simulink model "Scenario_3"  (R2020b)
settings: Solver=ode1  StartTime=0.0  StopTime=10.0  RelTol=1e-3
InitFcn:
  | Scenario_3_parameters;
values from neighbouring files (symbols this model uses):
  c0 = c0_zeb    (= 6.57988e-09)    [Scenario_17_parameters.m]    (also in Scenario_1_parameters.m = 6.37282e-09; Scenario_2_parameters.m = 6.37282e-09; Scenario_3_parameters.m)
  c0_hawk = 6.37282e-09    [Scenario_17_parameters.m]    (also in Scenario_1_parameters.m; Scenario_2_parameters.m; Scenario_3_parameters.m)
  c1 = c1_zeb    (= 9.15905e-09)    [Scenario_17_parameters.m]    (also in Scenario_1_parameters.m = 8.76156e-09; Scenario_2_parameters.m = 8.76156e-09; Scenario_3_parameters.m)
  c1_hawk = 8.76156e-09    [Scenario_17_parameters.m]    (also in Scenario_1_parameters.m; Scenario_2_parameters.m; Scenario_3_parameters.m)
  fg = 50    [Scenario_17_parameters.m]    (also in Scenario_1_parameters.m; Scenario_2_parameters.m; Scenario_3_parameters.m)
  G10gen = 0.85    [Scenario_3_parameters.m]
  G12gen = 0.85    [Scenario_3_parameters.m]
  G1gen = 0.50    (= 0.5)    [Scenario_17_parameters.m]    (also in Scenario_1_parameters.m = 0.2; Scenario_2_parameters.m = 0.1245; Scenario_3_parameters.m = 0.45)
  G2gen = 0.30    (= 0.3)    [Scenario_1_parameters.m]    (also in Scenario_2_parameters.m; Scenario_3_parameters.m = 0.4)
  G3gen = 0.25    [Scenario_1_parameters.m]    (also in Scenario_2_parameters.m = 0.2; Scenario_3_parameters.m = 0.6)
  G4gen = 0.95    [Scenario_3_parameters.m]
  G5gen = 0.75    [Scenario_17_parameters.m]    (also in Scenario_1_parameters.m = 0.22; Scenario_2_parameters.m = 0.2; Scenario_3_parameters.m = 0.7)
  G6gen = 0.90    (= 0.9)    [Scenario_17_parameters.m]    (also in Scenario_1_parameters.m = 0.41; Scenario_2_parameters.m = 0.2078; Scenario_3_parameters.m = 0.95)
  G7gen = 0.60    (= 0.6)    [Scenario_17_parameters.m]    (also in Scenario_1_parameters.m = 0.52; Scenario_2_parameters.m = 0.518; Scenario_3_parameters.m = 0.5)
  G8gen = 0.55    [Scenario_17_parameters.m]    (also in Scenario_3_parameters.m = 0.65)
  G9gen = 0.85    [Scenario_17_parameters.m]    (also in Scenario_3_parameters.m = 0.75)
  Ihvpk = Ihv*sqrt(2)    [Scenario_17_parameters.m]    (also in Scenario_1_parameters.m; Scenario_2_parameters.m; Scenario_3_parameters.m)
  l0 = l0_zeb    (= 0.00368)    [Scenario_17_parameters.m]    (also in Scenario_1_parameters.m = 0.00373; Scenario_2_parameters.m = 0.00373; Scenario_3_parameters.m)
  l0_hawk = 0.00373    [Scenario_17_parameters.m]    (also in Scenario_1_parameters.m; Scenario_2_parameters.m; Scenario_3_parameters.m)
  l1 = l1_zeb    (= 0.00128)    [Scenario_17_parameters.m]    (also in Scenario_1_parameters.m = 0.00133; Scenario_2_parameters.m = 0.00133; Scenario_3_parameters.m)
  L10dem = 0.10    (= 0.1)    [Scenario_3_parameters.m]
  L12dem = 0.025    [Scenario_17_parameters.m]    (also in Scenario_3_parameters.m = 0.005)
  L13dem = 0.005    [Scenario_3_parameters.m]
  l1_hawk = 0.00133    [Scenario_17_parameters.m]    (also in Scenario_1_parameters.m; Scenario_2_parameters.m; Scenario_3_parameters.m)
  L1dem = 0.25    [Scenario_17_parameters.m]    (also in Scenario_3_parameters.m = 0.1)
  L3dem = 0.30    (= 0.3)    [Scenario_17_parameters.m]    (also in Scenario_1_parameters.m = 0.1; Scenario_2_parameters.m = 0.1; Scenario_3_parameters.m = 0.2)
  L6dem = 0.15    [Scenario_1_parameters.m]    (also in Scenario_2_parameters.m; Scenario_3_parameters.m = 0.1)
  L7dem = 0.10    (= 0.1)    [Scenario_1_parameters.m]    (also in Scenario_2_parameters.m; Scenario_3_parameters.m = 0.15)
  L9dem = 0.15    [Scenario_17_parameters.m]    (also in Scenario_3_parameters.m)
  Pr = Sr*PF    (= 1900000000)    [Scenario_17_parameters.m]    (also in Scenario_1_parameters.m = 550050000; Scenario_2_parameters.m = 550050000; Scenario_3_parameters.m = 11640000000)
  Qr = sqrt(Sr^2 - Pr^2)    [Scenario_17_parameters.m]    (also in Scenario_1_parameters.m; Scenario_2_parameters.m; Scenario_3_parameters.m)
  r0 = r0_zeb    (= 0.39362)    [Scenario_17_parameters.m]    (also in Scenario_1_parameters.m = 0.44587; Scenario_2_parameters.m = 0.44587; Scenario_3_parameters.m)
  r0_hawk = 0.44587    [Scenario_17_parameters.m]    (also in Scenario_1_parameters.m; Scenario_2_parameters.m; Scenario_3_parameters.m)
  r1 = r1_zeb    (= 0.06862)    [Scenario_17_parameters.m]    (also in Scenario_1_parameters.m = 0.12087; Scenario_2_parameters.m = 0.12087; Scenario_3_parameters.m)
  r1_hawk = 0.12087    [Scenario_17_parameters.m]    (also in Scenario_1_parameters.m; Scenario_2_parameters.m; Scenario_3_parameters.m)
  Rtpu = Xtpu/40    (= 0.0025)    [Scenario_17_parameters.m]    (also in Scenario_1_parameters.m = 0.00375; Scenario_2_parameters.m = 0.00375; Scenario_3_parameters.m = 0.00375)
  S10non = 500e6    (= 500000000)    [Scenario_3_parameters.m]
  S12non = 1500e6    (= 1500000000)    [Scenario_3_parameters.m]
  S1non = 700e6    (= 700000000)    [Scenario_17_parameters.m]    (also in Scenario_1_parameters.m = 400000000; Scenario_2_parameters.m = 400000000; Scenario_3_parameters.m = 1000000000)
  S2non = 300e6    (= 300000000)    [Scenario_1_parameters.m]    (also in Scenario_2_parameters.m; Scenario_3_parameters.m = 3000000000)
  S3non = 200e6    (= 200000000)    [Scenario_1_parameters.m]    (also in Scenario_2_parameters.m; Scenario_3_parameters.m = 1000000000)
  S4non = 2000e6    (= 2000000000)    [Scenario_3_parameters.m]
  S5non = 400e6    (= 400000000)    [Scenario_17_parameters.m]    (also in Scenario_1_parameters.m = 500000000; Scenario_2_parameters.m = 500000000; Scenario_3_parameters.m = 2000000000)
  S6non = 150e6    (= 150000000)    [Scenario_17_parameters.m]    (also in Scenario_1_parameters.m = 400000000; Scenario_2_parameters.m = 400000000; Scenario_3_parameters.m = 3000000000)
  S7non = 1000e6    (= 1000000000)    [Scenario_17_parameters.m]    (also in Scenario_1_parameters.m = 200000000; Scenario_2_parameters.m = 200000000; Scenario_3_parameters.m = 4000000000)
  S8non = 600e6    (= 600000000)    [Scenario_17_parameters.m]    (also in Scenario_3_parameters.m = 2000000000)
  S9non = 200e6    (= 200000000)    [Scenario_17_parameters.m]    (also in Scenario_3_parameters.m = 1500000000)
  tonvsc = 0.01    [Scenario_17_parameters.m]    (also in Scenario_1_parameters.m = 0.02; Scenario_2_parameters.m; Scenario_3_parameters.m = 0.05)
  Ts = 100e-6    (= 0.0001)    [Scenario_17_parameters.m]    (also in Scenario_1_parameters.m; Scenario_2_parameters.m; Scenario_3_parameters.m = 5e-05)
  Vhv = 220e3    (= 220000)    [Scenario_17_parameters.m]    (also in Scenario_1_parameters.m; Scenario_2_parameters.m; Scenario_3_parameters.m)
  Vmv = 22e3    (= 22000)    [Scenario_17_parameters.m]    (also in Scenario_1_parameters.m; Scenario_2_parameters.m; Scenario_3_parameters.m)
  wc1 = wsw1/10    (= 848.230016469)    [Scenario_17_parameters.m]    (also in Scenario_1_parameters.m; Scenario_2_parameters.m; Scenario_3_parameters.m)
  wdc1 = wc1/10    (= 84.8230016469)    [Scenario_17_parameters.m]    (also in Scenario_1_parameters.m; Scenario_2_parameters.m; Scenario_3_parameters.m)
  wpq1 = wc1/10    (= 84.8230016469)    [Scenario_17_parameters.m]    (also in Scenario_1_parameters.m; Scenario_2_parameters.m; Scenario_3_parameters.m)
  wsw1 = ksw1*2*pi*fg    (= 8482.30016469)    [Scenario_17_parameters.m]    (also in Scenario_1_parameters.m; Scenario_2_parameters.m; Scenario_3_parameters.m)
  Xtpu = 0.10    (= 0.1)    [Scenario_17_parameters.m]    (also in Scenario_1_parameters.m = 0.15; Scenario_2_parameters.m = 0.15; Scenario_3_parameters.m = 0.15)
undefined symbols (not defined in the file or in its folder): D11, Delta, Kf, r, theta0
libraries: powerlib x426, simulink_extras x305, powerlib_meascontrol x139, pid_lib x109, eeGeneralControl x72, simulink x60, eeTransforms x54, spsFirstOrderFilterLib x36, eePwmGeneratorTwoLevel x9
(part 8 of 36)

== system Scenario_3/G10/VSC/VI measurement ==
  Current Measurement : powerlib/Measurements/Current Measurement  PhasorSimulation=on  OutputType=Complex  PSBequivalent=0
  Current Measurement1 : powerlib/Measurements/Current Measurement  PhasorSimulation=on  OutputType=Complex  PSBequivalent=0
  Current Measurement2 : powerlib/Measurements/Current Measurement  PhasorSimulation=on  OutputType=Complex  PSBequivalent=0
  Ground : powerlib/Elements/Ground  LConnTagsString=a
  Ground1 : powerlib/Elements/Ground  LConnTagsString=a
  Ground2 : powerlib/Elements/Ground  LConnTagsString=a
  Mux : Mux  Inputs=3
  Mux1 : Mux  Inputs=3
  Voltage Measurement : powerlib/Measurements/Voltage Measurement  PhasorSimulation=on  OutputType=Complex  PSBequivalent=0
  Voltage Measurement1 : powerlib/Measurements/Voltage Measurement  PhasorSimulation=on  OutputType=Complex  PSBequivalent=0
  Voltage Measurement2 : powerlib/Measurements/Voltage Measurement  PhasorSimulation=on  OutputType=Complex  PSBequivalent=0
  A : PMIOPort  Side=Left
  B : PMIOPort  Port=2  Side=Left
  C : PMIOPort  Port=3  Side=Left
  a : PMIOPort  Port=4  Side=Right
  b : PMIOPort  Port=5  Side=Right
  c : PMIOPort  Port=6  Side=Right
  Vs : Outport
  Is : Outport  Port=2
  wires:
  Mux1/1 -> Is/1
  Mux/1 -> Vs/1
  Voltage Measurement1/1 -> Mux/2
  Voltage Measurement2/1 -> Mux/3
  Current Measurement2/1 -> Mux1/3
  Voltage Measurement/1 -> Mux/1
  Current Measurement/1 -> Mux1/1
  Current Measurement1/1 -> Mux1/2
  connections:
  Voltage Measurement/LConn1 -- Current Measurement/LConn1 -- A/RConn1
  Current Measurement2/LConn1 -- C/RConn1 -- Voltage Measurement2/LConn1
  Current Measurement1/LConn1 -- Voltage Measurement1/LConn1 -- B/RConn1
  Current Measurement1/RConn1 -- b/RConn1
  Current Measurement/RConn1 -- a/RConn1
  Ground/LConn1 -- Voltage Measurement/LConn2
  Current Measurement2/RConn1 -- c/RConn1
  Ground1/LConn1 -- Voltage Measurement1/LConn2
  Ground2/LConn1 -- Voltage Measurement2/LConn2

== system Scenario_3/G10/VSC/VSC Control ==
  Block : Inport
  Vabc : Inport  Port=2
  Iabc : Inport  Port=3
  Pset : Inport  Port=4
  Qset : Inport  Port=5
  Control loops : Subsystem  Variant=on  VariantControlMode=label  LabelModeActiveChoice=Phasor_I_ref
  Measurements : Subsystem  Variant=on  VariantControlMode=label  LabelModeActiveChoice=Phasor
  Modulation : Subsystem  Variant=on  VariantControlMode=label  LabelModeActiveChoice=Phasor_I_and_PQ
  Mux : Mux  Inputs=2
  Ref : Outport
  m : Outport  Port=2
  wires:
  Control loops/2(iqd+-ref) -> Modulation/3(iqd+-*)
  Control loops/1(vqd+-ref) -> Modulation/2(vqd+-*)
  [PQabc] -> Mux/2
  Measurements/5(PQabc) -> [PQabc]
  Modulation/1(Ref) -> Ref/1
  Measurements/4(theta) -> [theta]
  Vabc/1 -> Measurements/1(Vabc)
  Measurements/1(vqd+-) -> Control loops/3(vqd+-), [vqdpn]
  Measurements/2(iqd+-) -> Control loops/4(iqd+-)
  Measurements/3(freq) -> Control loops/5(freq)
  [theta] -> Modulation/4(theta)
  [vqdpn] -> Modulation/1(vqd+-)
  Iabc/1 -> Measurements/2(Iabc)
  Mux/1 -> m/1
  Control loops/3(m) -> Mux/1
  Pset/1 -> Control loops/1(Pset)
  Qset/1 -> Control loops/2(Qset)
  Block/1 -> Control loops/6(Block)

== system Scenario_3/G10/VSC/VSC Model ==
  Ref : Inport
  EMT AVG : Subsystem  VariantControl=EMT_AVG
      settings: PortSchema="{\"entries\":[{\"content\":{\"sides\":[{\"content\":{\"connectorIds\":[\"LConn1\",\"LConn2\",\"LConn3\"]},\"type\":\"ConnectorPlacement.EquallySpacedRectSide\",\"uuid\":\"96043b84-a665-4cb2-a938-d6633d7ee474\"},{\"content\":{\"connectorIds\":[\"In1\"],\"side\":\"RIGHT\"},\"type\":\"ConnectorPlacement.EquallySpacedRectSide\",\"uuid\":\"064d463f-c23a-42ac-89ce-8dea3d446214\"},{\"content\":{\"connectorIds\":[],\"side\":\"TOP\"},\"type\":\"ConnectorPlacement.EquallySpacedRectSide\",\"uuid\":\"95ef669c-c6ed-44c3-8b69-447906728b6d\"}]},\"type\":\"ConnectorPlacement.EquallySpacedConnector\",\"uuid\":\"ea66db09-64d7-4d7e-ba7b-d769c56e2dbd\"}],\"packageUris\":[\"http://schema.mathworks.com/mf0/Connector/19700101\"],\"version\":\"1.0\"}"
  EMT SW : Subsystem  VariantControl=EMT_SW
      settings: PortSchema="{\"entries\":[{\"content\":{\"sides\":[{\"content\":{\"connectorIds\":[\"LConn1\",\"LConn2\",\"LConn3\"]},\"type\":\"ConnectorPlacement.EquallySpacedRectSide\",\"uuid\":\"96043b84-a665-4cb2-a938-d6633d7ee474\"},{\"content\":{\"connectorIds\":[\"In1\"],\"side\":\"RIGHT\"},\"type\":\"ConnectorPlacement.EquallySpacedRectSide\",\"uuid\":\"064d463f-c23a-42ac-89ce-8dea3d446214\"},{\"content\":{\"connectorIds\":[],\"side\":\"TOP\"},\"type\":\"ConnectorPlacement.EquallySpacedRectSide\",\"uuid\":\"95ef669c-c6ed-44c3-8b69-447906728b6d\"}]},\"type\":\"ConnectorPlacement.EquallySpacedConnector\",\"uuid\":\"ea66db09-64d7-4d7e-ba7b-d769c56e2dbd\"}],\"packageUris\":[\"http://schema.mathworks.com/mf0/Connector/19700101\"],\"version\":\"1.0\"}"
  Phasor : Subsystem  VariantControl=Phasor
      settings: PortSchema="{\"entries\":[{\"content\":{\"sides\":[{\"content\":{\"connectorIds\":[\"LConn1\",\"LConn2\",\"LConn3\"]},\"type\":\"ConnectorPlacement.EquallySpacedRectSide\",\"uuid\":\"96043b84-a665-4cb2-a938-d6633d7ee474\"},{\"content\":{\"connectorIds\":[\"In1\"],\"side\":\"RIGHT\"},\"type\":\"ConnectorPlacement.EquallySpacedRectSide\",\"uuid\":\"064d463f-c23a-42ac-89ce-8dea3d446214\"},{\"content\":{\"connectorIds\":[],\"side\":\"TOP\"},\"type\":\"ConnectorPlacement.EquallySpacedRectSide\",\"uuid\":\"95ef669c-c6ed-44c3-8b69-447906728b6d\"}]},\"type\":\"ConnectorPlacement.EquallySpacedConnector\",\"uuid\":\"ea66db09-64d7-4d7e-ba7b-d769c56e2dbd\"}],\"packageUris\":[\"http://schema.mathworks.com/mf0/Connector/19700101\"],\"version\":\"1.0\"}"
  A : PMIOPort  Side=Left
  B : PMIOPort  Port=2  Side=Left
  C : PMIOPort  Port=3  Side=Left

== system Scenario_3/G10/VSC/output signals ==
  Vs : Inport
  Is : Inport  Port=2
  control : Inport  Port=3
  Bus Creator : BusCreator  Inputs=15
  Demux : Demux  Outputs=13
  m : Outport
  wires:
  Bus Creator/1 -> m/1
  control/1 -> Demux/1
  Vs/1 -> Bus Creator/1  "Vabc"
  Is/1 -> Bus Creator/2  "Iabc"
  Demux/1 -> Bus Creator/3  "vqp"
  Demux/2 -> Bus Creator/4  "vdp"
  Demux/3 -> Bus Creator/5  "vqn"
  Demux/4 -> Bus Creator/6  "vdn"
  Demux/5 -> Bus Creator/7  "iqp"
  Demux/6 -> Bus Creator/8  "idp"
  Demux/7 -> Bus Creator/9  "iqn"
  Demux/8 -> Bus Creator/10  "idn"
  Demux/9 -> Bus Creator/11  "f"
  Demux/10 -> Bus Creator/12  "Pdq"
  Demux/11 -> Bus Creator/13  "Qdq"
  Demux/12 -> Bus Creator/14  "Pabc"
  Demux/13 -> Bus Creator/15  "Qabc"

== system Scenario_3/G12/VSC/VI measurement ==
  Current Measurement : powerlib/Measurements/Current Measurement  PhasorSimulation=on  OutputType=Complex  PSBequivalent=0
  Current Measurement1 : powerlib/Measurements/Current Measurement  PhasorSimulation=on  OutputType=Complex  PSBequivalent=0
  Current Measurement2 : powerlib/Measurements/Current Measurement  PhasorSimulation=on  OutputType=Complex  PSBequivalent=0
  Ground : powerlib/Elements/Ground  LConnTagsString=a
  Ground1 : powerlib/Elements/Ground  LConnTagsString=a
  Ground2 : powerlib/Elements/Ground  LConnTagsString=a
  Mux : Mux  Inputs=3
  Mux1 : Mux  Inputs=3
  Voltage Measurement : powerlib/Measurements/Voltage Measurement  PhasorSimulation=on  OutputType=Complex  PSBequivalent=0
  Voltage Measurement1 : powerlib/Measurements/Voltage Measurement  PhasorSimulation=on  OutputType=Complex  PSBequivalent=0
  Voltage Measurement2 : powerlib/Measurements/Voltage Measurement  PhasorSimulation=on  OutputType=Complex  PSBequivalent=0
  A : PMIOPort  Side=Left
  B : PMIOPort  Port=2  Side=Left
  C : PMIOPort  Port=3  Side=Left
  a : PMIOPort  Port=4  Side=Right
  b : PMIOPort  Port=5  Side=Right
  c : PMIOPort  Port=6  Side=Right
  Vs : Outport
  Is : Outport  Port=2
  wires:
  Mux1/1 -> Is/1
  Mux/1 -> Vs/1
  Voltage Measurement1/1 -> Mux/2
  Voltage Measurement2/1 -> Mux/3
  Current Measurement2/1 -> Mux1/3
  Voltage Measurement/1 -> Mux/1
  Current Measurement/1 -> Mux1/1
  Current Measurement1/1 -> Mux1/2
  connections:
  Voltage Measurement/LConn1 -- Current Measurement/LConn1 -- A/RConn1
  Current Measurement2/LConn1 -- C/RConn1 -- Voltage Measurement2/LConn1
  Current Measurement1/LConn1 -- Voltage Measurement1/LConn1 -- B/RConn1
  Current Measurement1/RConn1 -- b/RConn1
  Current Measurement/RConn1 -- a/RConn1
  Ground/LConn1 -- Voltage Measurement/LConn2
  Current Measurement2/RConn1 -- c/RConn1
  Ground1/LConn1 -- Voltage Measurement1/LConn2
  Ground2/LConn1 -- Voltage Measurement2/LConn2

== system Scenario_3/G12/VSC/VSC Control ==
  Block : Inport
  Vabc : Inport  Port=2
  Iabc : Inport  Port=3
  Pset : Inport  Port=4
  Qset : Inport  Port=5
  Control loops : Subsystem  Variant=on  VariantControlMode=label  LabelModeActiveChoice=Phasor_I_ref
  Measurements : Subsystem  Variant=on  VariantControlMode=label  LabelModeActiveChoice=Phasor
  Modulation : Subsystem  Variant=on  VariantControlMode=label  LabelModeActiveChoice=Phasor_I_and_PQ
  Mux : Mux  Inputs=2
  Ref : Outport
  m : Outport  Port=2
  wires:
  Control loops/2(iqd+-ref) -> Modulation/3(iqd+-*)
  Control loops/1(vqd+-ref) -> Modulation/2(vqd+-*)
  [PQabc] -> Mux/2
  Measurements/5(PQabc) -> [PQabc]
  Modulation/1(Ref) -> Ref/1
  Measurements/4(theta) -> [theta]
  Vabc/1 -> Measurements/1(Vabc)
  Measurements/1(vqd+-) -> Control loops/3(vqd+-), [vqdpn]
  Measurements/2(iqd+-) -> Control loops/4(iqd+-)
  Measurements/3(freq) -> Control loops/5(freq)
  [theta] -> Modulation/4(theta)
  [vqdpn] -> Modulation/1(vqd+-)
  Iabc/1 -> Measurements/2(Iabc)
  Mux/1 -> m/1
  Control loops/3(m) -> Mux/1
  Pset/1 -> Control loops/1(Pset)
  Qset/1 -> Control loops/2(Qset)
  Block/1 -> Control loops/6(Block)

== system Scenario_3/G12/VSC/VSC Model ==
  Ref : Inport
  EMT AVG : Subsystem  VariantControl=EMT_AVG
      settings: PortSchema="{\"entries\":[{\"content\":{\"sides\":[{\"content\":{\"connectorIds\":[\"LConn1\",\"LConn2\",\"LConn3\"]},\"type\":\"ConnectorPlacement.EquallySpacedRectSide\",\"uuid\":\"96043b84-a665-4cb2-a938-d6633d7ee474\"},{\"content\":{\"connectorIds\":[\"In1\"],\"side\":\"RIGHT\"},\"type\":\"ConnectorPlacement.EquallySpacedRectSide\",\"uuid\":\"064d463f-c23a-42ac-89ce-8dea3d446214\"},{\"content\":{\"connectorIds\":[],\"side\":\"TOP\"},\"type\":\"ConnectorPlacement.EquallySpacedRectSide\",\"uuid\":\"95ef669c-c6ed-44c3-8b69-447906728b6d\"}]},\"type\":\"ConnectorPlacement.EquallySpacedConnector\",\"uuid\":\"ea66db09-64d7-4d7e-ba7b-d769c56e2dbd\"}],\"packageUris\":[\"http://schema.mathworks.com/mf0/Connector/19700101\"],\"version\":\"1.0\"}"
  EMT SW : Subsystem  VariantControl=EMT_SW
      settings: PortSchema="{\"entries\":[{\"content\":{\"sides\":[{\"content\":{\"connectorIds\":[\"LConn1\",\"LConn2\",\"LConn3\"]},\"type\":\"ConnectorPlacement.EquallySpacedRectSide\",\"uuid\":\"96043b84-a665-4cb2-a938-d6633d7ee474\"},{\"content\":{\"connectorIds\":[\"In1\"],\"side\":\"RIGHT\"},\"type\":\"ConnectorPlacement.EquallySpacedRectSide\",\"uuid\":\"064d463f-c23a-42ac-89ce-8dea3d446214\"},{\"content\":{\"connectorIds\":[],\"side\":\"TOP\"},\"type\":\"ConnectorPlacement.EquallySpacedRectSide\",\"uuid\":\"95ef669c-c6ed-44c3-8b69-447906728b6d\"}]},\"type\":\"ConnectorPlacement.EquallySpacedConnector\",\"uuid\":\"ea66db09-64d7-4d7e-ba7b-d769c56e2dbd\"}],\"packageUris\":[\"http://schema.mathworks.com/mf0/Connector/19700101\"],\"version\":\"1.0\"}"
  Phasor : Subsystem  VariantControl=Phasor
      settings: PortSchema="{\"entries\":[{\"content\":{\"sides\":[{\"content\":{\"connectorIds\":[\"LConn1\",\"LConn2\",\"LConn3\"]},\"type\":\"ConnectorPlacement.EquallySpacedRectSide\",\"uuid\":\"96043b84-a665-4cb2-a938-d6633d7ee474\"},{\"content\":{\"connectorIds\":[\"In1\"],\"side\":\"RIGHT\"},\"type\":\"ConnectorPlacement.EquallySpacedRectSide\",\"uuid\":\"064d463f-c23a-42ac-89ce-8dea3d446214\"},{\"content\":{\"connectorIds\":[],\"side\":\"TOP\"},\"type\":\"ConnectorPlacement.EquallySpacedRectSide\",\"uuid\":\"95ef669c-c6ed-44c3-8b69-447906728b6d\"}]},\"type\":\"ConnectorPlacement.EquallySpacedConnector\",\"uuid\":\"ea66db09-64d7-4d7e-ba7b-d769c56e2dbd\"}],\"packageUris\":[\"http://schema.mathworks.com/mf0/Connector/19700101\"],\"version\":\"1.0\"}"
  A : PMIOPort  Side=Left
  B : PMIOPort  Port=2  Side=Left
  C : PMIOPort  Port=3  Side=Left

== system Scenario_3/G12/VSC/output signals ==
  Vs : Inport
  Is : Inport  Port=2
  control : Inport  Port=3
  Bus Creator : BusCreator  Inputs=15
  Demux : Demux  Outputs=13
  m : Outport
  wires:
  Bus Creator/1 -> m/1
  control/1 -> Demux/1
  Vs/1 -> Bus Creator/1  "Vabc"
  Is/1 -> Bus Creator/2  "Iabc"
  Demux/1 -> Bus Creator/3  "vqp"
  Demux/2 -> Bus Creator/4  "vdp"
  Demux/3 -> Bus Creator/5  "vqn"
  Demux/4 -> Bus Creator/6  "vdn"
  Demux/5 -> Bus Creator/7  "iqp"
  Demux/6 -> Bus Creator/8  "idp"
  Demux/7 -> Bus Creator/9  "iqn"
  Demux/8 -> Bus Creator/10  "idn"
  Demux/9 -> Bus Creator/11  "f"
  Demux/10 -> Bus Creator/12  "Pdq"
  Demux/11 -> Bus Creator/13  "Qdq"
  Demux/12 -> Bus Creator/14  "Pabc"
  Demux/13 -> Bus Creator/15  "Qabc"

== system Scenario_3/G2/Exciter System/PSS ==
  note: Power System Stabilizer (PSS2A)
  dw : Inport
  Pgen : Inport  Port=2
  Gain : Gain  Gain=Ks1
  Gain1 : Gain  Gain=Ks3
  Saturation : Saturate  UpperLimit=Vstmax  LowerLimit=Vstmin
  Sum1 : Sum  Inputs=|++
  Sum2 : Sum  Inputs=|+-
  Transfer Fcn1 : TransferFcn  Numerator=[Tw1 0]  Denominator=[Tw1 1]
  Transfer Fcn2 : TransferFcn  Numerator=[Tw3 0]  Denominator=[Tw3 1]
  Transfer Fcn3 : TransferFcn  Numerator=[Tw2 0]  Denominator=[Tw2 1]
  Transfer Fcn4 : TransferFcn  Denominator=[T6 1]
  Transfer Fcn5 : TransferFcn  Numerator=[T8 1].^N  Denominator=[T9 1].^(M*N)
  Transfer Fcn6 : TransferFcn  Numerator=[T1 1]  Denominator=[T2 1]
  Transfer Fcn7 : TransferFcn  Numerator=[T3 1]  Denominator=[T4 1]
  Transfer Fcn8 : TransferFcn  Numerator=[Tw4 0]  Denominator=[Tw4 1]
  Transfer Fcn9 : TransferFcn  Numerator=[Ks2]  Denominator=[T7 1]
  Vothsg : Outport
  wires:
  Transfer Fcn9/1 -> Sum2/2, Gain1/1
  Gain1/1 -> Sum1/2
  Transfer Fcn8/1 -> Transfer Fcn9/1
  Transfer Fcn2/1 -> Transfer Fcn8/1
  Pgen/1 -> Transfer Fcn2/1
  Saturation/1 -> Vothsg/1
  Transfer Fcn7/1 -> Saturation/1
  Transfer Fcn6/1 -> Transfer Fcn7/1
  Gain/1 -> Transfer Fcn6/1
  Sum2/1 -> Gain/1
  Transfer Fcn5/1 -> Sum2/1
  Sum1/1 -> Transfer Fcn5/1
  Transfer Fcn4/1 -> Sum1/1
  Transfer Fcn3/1 -> Transfer Fcn4/1
  Transfer Fcn1/1 -> Transfer Fcn3/1
  dw/1 -> Transfer Fcn1/1

== system Scenario_3/G2/Exciter System/SEXS ==
  note: The controller parameters provided by ENTSO-E
      | define different names for the parameters:
      |
      | ENTSO-E = IEEE Std 421.5-2005
      | Ta = Tc
      | Tb = Tb
      | K = Ka
      | Te = Ta
      | Emax = Vrmax
      | Emin = Vrmin
  note: The exciter model provided by ENTSO-E most similar to the IEEE is the Type AC4A excitation system model
  Vref : Inport
  Vc : Inport  Port=2
  Vs : Inport  Port=3
  1st ord transfer fcn windup limiter : Subsystem  mask{Gain=K, tau=Te, Vmax=Emax, Vmin=Emin, y0=Vf0}
      mask prompts: tau "Time constant"; y0 "Initial output"
  Constant : Constant  Value=Vf0/K
  Saturation : Saturate  Commented=through  UpperLimit=0.1  LowerLimit=-0.1
  Sum : Sum  Inputs=+-+
  Sum1 : Sum  Inputs=|++
  Transfer Fcn (with initial outputs)1 : simulink_extras/Additional Linear/Transfer Fcn (with initial outputs)  N=[Ta 1]  D=[Tb 1]  Y0=Vf0/K  U0=Vf0/K
  Efd : Outport
  wires:
  1st ord transfer fcn windup limiter/1(Out1) -> Efd/1
  Vs/1 -> Sum/3
  Vref/1 -> Sum/1
  Vc/1 -> Sum/2
  Transfer Fcn (with initial outputs)1/1 -> 1st ord transfer fcn windup limiter/1(In1)
  Saturation/1 -> Transfer Fcn (with initial outputs)1/1
  Sum/1 -> Sum1/1
  Sum1/1 -> Saturation/1
  Constant/1 -> Sum1/2

== system Scenario_3/G2/Exciter System/TR and LC_test ==
  note: Rc and Xc should be negative values in case of voltage regulated after an impedance
  note: Fig 4.1 of IEEE Std 421.5-2005
  note: Vt and It should be phasors (complex quantities)
  note: compensated
      | impedance
  note: Terminal voltage transducer and optional load compensation
  Vt : Inport
  It : Inport  Port=2
  Abs : Abs
  Abs1 : Abs
  Rc+jXc : Gain  Gain=abs(Rc+1i*Xc)
  Saturation : Saturate  UpperLimit=1.2  LowerLimit=0.8
  Sum : Sum  Inputs=|+-
  Transfer Fcn (with initial outputs) : simulink_extras/Additional Linear/Transfer Fcn (with initial outputs)  N=[1]  D=[Tr 1]  Y0=1  U0=1
  Vc : Outport
  wires:
  Abs1/1 -> Rc+jXc/1
  Abs/1 -> Sum/1
  It/1 -> Abs1/1
  Sum/1 -> Transfer Fcn (with initial outputs)/1
  Rc+jXc/1 -> Sum/2
  Transfer Fcn (with initial outputs)/1 -> Saturation/1
  Vt/1 -> Abs/1
  Saturation/1 -> Vc/1

== system Scenario_3/G3/Exciter System/PSS1 ==
  note: Power System Stabilizer (PSS2A)
  dw : Inport
  Pgen : Inport  Port=2
  Gain : Gain  Gain=Ks1
  Gain1 : Gain  Gain=Ks3
  Saturation : Saturate  UpperLimit=Vstmax  LowerLimit=Vstmin
  Sum1 : Sum  Inputs=|++
  Sum2 : Sum  Inputs=|+-
  Transfer Fcn1 : TransferFcn  Numerator=[Tw1 0]  Denominator=[Tw1 1]
  Transfer Fcn2 : TransferFcn  Numerator=[Tw3 0]  Denominator=[Tw3 1]
  Transfer Fcn3 : TransferFcn  Numerator=[Tw2 0]  Denominator=[Tw2 1]
  Transfer Fcn4 : TransferFcn  Denominator=[T6 1]
  Transfer Fcn5 : TransferFcn  Numerator=[T8 1].^N  Denominator=[T9 1].^(M*N)
  Transfer Fcn6 : TransferFcn  Numerator=[T1 1]  Denominator=[T2 1]
  Transfer Fcn7 : TransferFcn  Numerator=[T3 1]  Denominator=[T4 1]
  Transfer Fcn8 : TransferFcn  Numerator=[Tw4 0]  Denominator=[Tw4 1]
  Transfer Fcn9 : TransferFcn  Numerator=[Ks2]  Denominator=[T7 1]
  Vothsg : Outport
  wires:
  dw/1 -> Transfer Fcn1/1
  Transfer Fcn1/1 -> Transfer Fcn3/1
  Transfer Fcn3/1 -> Transfer Fcn4/1
  Transfer Fcn4/1 -> Sum1/1
  Sum1/1 -> Transfer Fcn5/1
  Transfer Fcn5/1 -> Sum2/1
  Sum2/1 -> Gain/1
  Gain/1 -> Transfer Fcn6/1
  Transfer Fcn6/1 -> Transfer Fcn7/1
  Transfer Fcn7/1 -> Saturation/1
  Saturation/1 -> Vothsg/1
  Pgen/1 -> Transfer Fcn2/1
  Transfer Fcn2/1 -> Transfer Fcn8/1
  Transfer Fcn8/1 -> Transfer Fcn9/1
  Gain1/1 -> Sum1/2
  Transfer Fcn9/1 -> Gain1/1, Sum2/2

== system Scenario_3/G3/Exciter System/SEXS ==
  note: The controller parameters provided by ENTSO-E
      | define different names for the parameters:
      |
      | ENTSO-E = IEEE Std 421.5-2005
      | Ta = Tc
      | Tb = Tb
      | K = Ka
      | Te = Ta
      | Emax = Vrmax
      | Emin = Vrmin
  note: The exciter model provided by ENTSO-E most similar to the IEEE is the Type AC4A excitation system model
  Vref : Inport
  Vc : Inport  Port=2
  Vs : Inport  Port=3
  1st ord transfer fcn windup limiter : Subsystem  mask{Gain=K, tau=Te, Vmax=Emax, Vmin=Emin, y0=Vf0}
      mask prompts: tau "Time constant"; y0 "Initial output"
  Constant : Constant  Value=Vf0/K
  Saturation : Saturate  Commented=through  UpperLimit=0.1  LowerLimit=-0.1
  Sum : Sum  Inputs=+-+
  Sum1 : Sum  Inputs=|++
  Transfer Fcn (with initial outputs)1 : simulink_extras/Additional Linear/Transfer Fcn (with initial outputs)  N=[Ta 1]  D=[Tb 1]  Y0=Vf0/K  U0=Vf0/K
  Efd : Outport
  wires:
  1st ord transfer fcn windup limiter/1(Out1) -> Efd/1
  Vs/1 -> Sum/3
  Vref/1 -> Sum/1
  Vc/1 -> Sum/2
  Transfer Fcn (with initial outputs)1/1 -> 1st ord transfer fcn windup limiter/1(In1)
  Saturation/1 -> Transfer Fcn (with initial outputs)1/1
  Sum/1 -> Sum1/1
  Sum1/1 -> Saturation/1
  Constant/1 -> Sum1/2

== system Scenario_3/G3/Exciter System/TR and LC_test ==
  note: Terminal voltage transducer and optional load compensation
  note: compensated
      | impedance
  note: Vt and It should be phasors (complex quantities)
  note: Fig 4.1 of IEEE Std 421.5-2005
  note: Rc and Xc should be negative values in case of voltage regulated after an impedance
  Vt : Inport
  It : Inport  Port=2
  Abs : Abs
  Abs1 : Abs
  Rc+jXc : Gain  Gain=abs(Rc+1i*Xc)
  Saturation : Saturate  UpperLimit=1.2  LowerLimit=0.8
  Sum : Sum  Inputs=|+-
  Transfer Fcn (with initial outputs) : simulink_extras/Additional Linear/Transfer Fcn (with initial outputs)  Commented=through  N=[1]  D=[Tr 1]  Y0=1  U0=1
  Vc : Outport
  wires:
  Saturation/1 -> Vc/1
  Vt/1 -> Abs/1
  Transfer Fcn (with initial outputs)/1 -> Saturation/1
  Rc+jXc/1 -> Sum/2
  Sum/1 -> Transfer Fcn (with initial outputs)/1
  It/1 -> Abs1/1
  Abs/1 -> Sum/1
  Abs1/1 -> Rc+jXc/1

== system Scenario_3/G4/VSC/VI measurement ==
  Current Measurement : powerlib/Measurements/Current Measurement  PhasorSimulation=on  OutputType=Complex  PSBequivalent=0
  Current Measurement1 : powerlib/Measurements/Current Measurement  PhasorSimulation=on  OutputType=Complex  PSBequivalent=0
  Current Measurement2 : powerlib/Measurements/Current Measurement  PhasorSimulation=on  OutputType=Complex  PSBequivalent=0
  Ground : powerlib/Elements/Ground  LConnTagsString=a
  Ground1 : powerlib/Elements/Ground  LConnTagsString=a
  Ground2 : powerlib/Elements/Ground  LConnTagsString=a
  Mux : Mux  Inputs=3
  Mux1 : Mux  Inputs=3
  Voltage Measurement : powerlib/Measurements/Voltage Measurement  PhasorSimulation=on  OutputType=Complex  PSBequivalent=0
  Voltage Measurement1 : powerlib/Measurements/Voltage Measurement  PhasorSimulation=on  OutputType=Complex  PSBequivalent=0
  Voltage Measurement2 : powerlib/Measurements/Voltage Measurement  PhasorSimulation=on  OutputType=Complex  PSBequivalent=0
  A : PMIOPort  Side=Left
  B : PMIOPort  Port=2  Side=Left
  C : PMIOPort  Port=3  Side=Left
  a : PMIOPort  Port=4  Side=Right
  b : PMIOPort  Port=5  Side=Right
  c : PMIOPort  Port=6  Side=Right
  Vs : Outport
  Is : Outport  Port=2
  wires:
  Mux1/1 -> Is/1
  Mux/1 -> Vs/1
  Voltage Measurement1/1 -> Mux/2
  Voltage Measurement2/1 -> Mux/3
  Current Measurement2/1 -> Mux1/3
  Voltage Measurement/1 -> Mux/1
  Current Measurement/1 -> Mux1/1
  Current Measurement1/1 -> Mux1/2
  connections:
  Voltage Measurement/LConn1 -- Current Measurement/LConn1 -- A/RConn1
  Current Measurement2/LConn1 -- C/RConn1 -- Voltage Measurement2/LConn1
  Current Measurement1/LConn1 -- Voltage Measurement1/LConn1 -- B/RConn1
  Current Measurement1/RConn1 -- b/RConn1
  Current Measurement/RConn1 -- a/RConn1
  Ground/LConn1 -- Voltage Measurement/LConn2
  Current Measurement2/RConn1 -- c/RConn1
  Ground1/LConn1 -- Voltage Measurement1/LConn2
  Ground2/LConn1 -- Voltage Measurement2/LConn2

== system Scenario_3/G4/VSC/VSC Control ==
  Block : Inport
  Vabc : Inport  Port=2
  Iabc : Inport  Port=3
  Pset : Inport  Port=4
  Qset : Inport  Port=5
  Control loops : Subsystem  Variant=on  VariantControlMode=label  LabelModeActiveChoice=Phasor_I_ref
  Measurements : Subsystem  Variant=on  VariantControlMode=label  LabelModeActiveChoice=Phasor
  Modulation : Subsystem  Variant=on  VariantControlMode=label  LabelModeActiveChoice=Phasor_I_and_PQ
  Mux : Mux  Inputs=2
  Ref : Outport
  m : Outport  Port=2
  wires:
  Control loops/2(iqd+-ref) -> Modulation/3(iqd+-*)
  Control loops/1(vqd+-ref) -> Modulation/2(vqd+-*)
  [PQabc] -> Mux/2
  Measurements/5(PQabc) -> [PQabc]
  Modulation/1(Ref) -> Ref/1
  Measurements/4(theta) -> [theta]
  Vabc/1 -> Measurements/1(Vabc)
  Measurements/1(vqd+-) -> Control loops/3(vqd+-), [vqdpn]
  Measurements/2(iqd+-) -> Control loops/4(iqd+-)
  Measurements/3(freq) -> Control loops/5(freq)
  [theta] -> Modulation/4(theta)
  [vqdpn] -> Modulation/1(vqd+-)
  Iabc/1 -> Measurements/2(Iabc)
  Mux/1 -> m/1
  Control loops/3(m) -> Mux/1
  Pset/1 -> Control loops/1(Pset)
  Qset/1 -> Control loops/2(Qset)
  Block/1 -> Control loops/6(Block)

== system Scenario_3/G4/VSC/VSC Model ==
  Ref : Inport
  EMT AVG : Subsystem  VariantControl=EMT_AVG
      settings: PortSchema="{\"entries\":[{\"content\":{\"sides\":[{\"content\":{\"connectorIds\":[\"LConn1\",\"LConn2\",\"LConn3\"]},\"type\":\"ConnectorPlacement.EquallySpacedRectSide\",\"uuid\":\"96043b84-a665-4cb2-a938-d6633d7ee474\"},{\"content\":{\"connectorIds\":[\"In1\"],\"side\":\"RIGHT\"},\"type\":\"ConnectorPlacement.EquallySpacedRectSide\",\"uuid\":\"064d463f-c23a-42ac-89ce-8dea3d446214\"},{\"content\":{\"connectorIds\":[],\"side\":\"TOP\"},\"type\":\"ConnectorPlacement.EquallySpacedRectSide\",\"uuid\":\"95ef669c-c6ed-44c3-8b69-447906728b6d\"}]},\"type\":\"ConnectorPlacement.EquallySpacedConnector\",\"uuid\":\"ea66db09-64d7-4d7e-ba7b-d769c56e2dbd\"}],\"packageUris\":[\"http://schema.mathworks.com/mf0/Connector/19700101\"],\"version\":\"1.0\"}"
  EMT SW : Subsystem  VariantControl=EMT_SW
      settings: PortSchema="{\"entries\":[{\"content\":{\"sides\":[{\"content\":{\"connectorIds\":[\"LConn1\",\"LConn2\",\"LConn3\"]},\"type\":\"ConnectorPlacement.EquallySpacedRectSide\",\"uuid\":\"96043b84-a665-4cb2-a938-d6633d7ee474\"},{\"content\":{\"connectorIds\":[\"In1\"],\"side\":\"RIGHT\"},\"type\":\"ConnectorPlacement.EquallySpacedRectSide\",\"uuid\":\"064d463f-c23a-42ac-89ce-8dea3d446214\"},{\"content\":{\"connectorIds\":[],\"side\":\"TOP\"},\"type\":\"ConnectorPlacement.EquallySpacedRectSide\",\"uuid\":\"95ef669c-c6ed-44c3-8b69-447906728b6d\"}]},\"type\":\"ConnectorPlacement.EquallySpacedConnector\",\"uuid\":\"ea66db09-64d7-4d7e-ba7b-d769c56e2dbd\"}],\"packageUris\":[\"http://schema.mathworks.com/mf0/Connector/19700101\"],\"version\":\"1.0\"}"
  Phasor : Subsystem  VariantControl=Phasor
      settings: PortSchema="{\"entries\":[{\"content\":{\"sides\":[{\"content\":{\"connectorIds\":[\"LConn1\",\"LConn2\",\"LConn3\"]},\"type\":\"ConnectorPlacement.EquallySpacedRectSide\",\"uuid\":\"96043b84-a665-4cb2-a938-d6633d7ee474\"},{\"content\":{\"connectorIds\":[\"In1\"],\"side\":\"RIGHT\"},\"type\":\"ConnectorPlacement.EquallySpacedRectSide\",\"uuid\":\"064d463f-c23a-42ac-89ce-8dea3d446214\"},{\"content\":{\"connectorIds\":[],\"side\":\"TOP\"},\"type\":\"ConnectorPlacement.EquallySpacedRectSide\",\"uuid\":\"95ef669c-c6ed-44c3-8b69-447906728b6d\"}]},\"type\":\"ConnectorPlacement.EquallySpacedConnector\",\"uuid\":\"ea66db09-64d7-4d7e-ba7b-d769c56e2dbd\"}],\"packageUris\":[\"http://schema.mathworks.com/mf0/Connector/19700101\"],\"version\":\"1.0\"}"
  A : PMIOPort  Side=Left
  B : PMIOPort  Port=2  Side=Left
  C : PMIOPort  Port=3  Side=Left

== system Scenario_3/G4/VSC/output signals ==
  Vs : Inport
  Is : Inport  Port=2
  control : Inport  Port=3
  Bus Creator : BusCreator  Inputs=15
  Demux : Demux  Outputs=13
  m : Outport
  wires:
  Bus Creator/1 -> m/1
  control/1 -> Demux/1
  Vs/1 -> Bus Creator/1  "Vabc"
  Is/1 -> Bus Creator/2  "Iabc"
  Demux/1 -> Bus Creator/3  "vqp"
  Demux/2 -> Bus Creator/4  "vdp"
  Demux/3 -> Bus Creator/5  "vqn"
  Demux/4 -> Bus Creator/6  "vdn"
  Demux/5 -> Bus Creator/7  "iqp"
  Demux/6 -> Bus Creator/8  "idp"
  Demux/7 -> Bus Creator/9  "iqn"
  Demux/8 -> Bus Creator/10  "idn"
  Demux/9 -> Bus Creator/11  "f"
  Demux/10 -> Bus Creator/12  "Pdq"
  Demux/11 -> Bus Creator/13  "Qdq"
  Demux/12 -> Bus Creator/14  "Pabc"
  Demux/13 -> Bus Creator/15  "Qabc"

== system Scenario_3/G6/VSC/VI measurement ==
  Current Measurement : powerlib/Measurements/Current Measurement  PhasorSimulation=on  OutputType=Complex  PSBequivalent=0
  Current Measurement1 : powerlib/Measurements/Current Measurement  PhasorSimulation=on  OutputType=Complex  PSBequivalent=0
  Current Measurement2 : powerlib/Measurements/Current Measurement  PhasorSimulation=on  OutputType=Complex  PSBequivalent=0
  Ground : powerlib/Elements/Ground  LConnTagsString=a
  Ground1 : powerlib/Elements/Ground  LConnTagsString=a
  Ground2 : powerlib/Elements/Ground  LConnTagsString=a
  Mux : Mux  Inputs=3
  Mux1 : Mux  Inputs=3
  Voltage Measurement : powerlib/Measurements/Voltage Measurement  PhasorSimulation=on  OutputType=Complex  PSBequivalent=0
  Voltage Measurement1 : powerlib/Measurements/Voltage Measurement  PhasorSimulation=on  OutputType=Complex  PSBequivalent=0
  Voltage Measurement2 : powerlib/Measurements/Voltage Measurement  PhasorSimulation=on  OutputType=Complex  PSBequivalent=0
  A : PMIOPort  Side=Left
  B : PMIOPort  Port=2  Side=Left
  C : PMIOPort  Port=3  Side=Left
  a : PMIOPort  Port=4  Side=Right
  b : PMIOPort  Port=5  Side=Right
  c : PMIOPort  Port=6  Side=Right
  Vs : Outport
  Is : Outport  Port=2
  wires:
  Mux1/1 -> Is/1
  Mux/1 -> Vs/1
  Voltage Measurement1/1 -> Mux/2
  Voltage Measurement2/1 -> Mux/3
  Current Measurement2/1 -> Mux1/3
  Voltage Measurement/1 -> Mux/1
  Current Measurement/1 -> Mux1/1
  Current Measurement1/1 -> Mux1/2
  connections:
  Voltage Measurement/LConn1 -- Current Measurement/LConn1 -- A/RConn1
  Current Measurement2/LConn1 -- C/RConn1 -- Voltage Measurement2/LConn1
  Current Measurement1/LConn1 -- Voltage Measurement1/LConn1 -- B/RConn1
  Current Measurement1/RConn1 -- b/RConn1
  Current Measurement/RConn1 -- a/RConn1
  Ground/LConn1 -- Voltage Measurement/LConn2
  Current Measurement2/RConn1 -- c/RConn1
  Ground1/LConn1 -- Voltage Measurement1/LConn2
  Ground2/LConn1 -- Voltage Measurement2/LConn2

== system Scenario_3/G6/VSC/VSC Control ==
  Block : Inport
  Vabc : Inport  Port=2
  Iabc : Inport  Port=3
  Pset : Inport  Port=4
  Qset : Inport  Port=5
  Control loops : Subsystem  Variant=on  VariantControlMode=label  LabelModeActiveChoice=Phasor_I_ref
  Measurements : Subsystem  Variant=on  VariantControlMode=label  LabelModeActiveChoice=Phasor
  Modulation : Subsystem  Variant=on  VariantControlMode=label  LabelModeActiveChoice=Phasor_I_and_PQ
  Mux : Mux  Inputs=2
  Ref : Outport
  m : Outport  Port=2
  wires:
  Control loops/2(iqd+-ref) -> Modulation/3(iqd+-*)
  Control loops/1(vqd+-ref) -> Modulation/2(vqd+-*)
  [PQabc] -> Mux/2
  Measurements/5(PQabc) -> [PQabc]
  Modulation/1(Ref) -> Ref/1
  Measurements/4(theta) -> [theta]
  Vabc/1 -> Measurements/1(Vabc)
  Measurements/1(vqd+-) -> Control loops/3(vqd+-), [vqdpn]
  Measurements/2(iqd+-) -> Control loops/4(iqd+-)
  Measurements/3(freq) -> Control loops/5(freq)
  [theta] -> Modulation/4(theta)
  [vqdpn] -> Modulation/1(vqd+-)
  Iabc/1 -> Measurements/2(Iabc)
  Mux/1 -> m/1
  Control loops/3(m) -> Mux/1
  Pset/1 -> Control loops/1(Pset)
  Qset/1 -> Control loops/2(Qset)
  Block/1 -> Control loops/6(Block)

== system Scenario_3/G6/VSC/VSC Model ==
  Ref : Inport
  EMT AVG : Subsystem  VariantControl=EMT_AVG
      settings: PortSchema="{\"entries\":[{\"content\":{\"sides\":[{\"content\":{\"connectorIds\":[\"LConn1\",\"LConn2\",\"LConn3\"]},\"type\":\"ConnectorPlacement.EquallySpacedRectSide\",\"uuid\":\"96043b84-a665-4cb2-a938-d6633d7ee474\"},{\"content\":{\"connectorIds\":[\"In1\"],\"side\":\"RIGHT\"},\"type\":\"ConnectorPlacement.EquallySpacedRectSide\",\"uuid\":\"064d463f-c23a-42ac-89ce-8dea3d446214\"},{\"content\":{\"connectorIds\":[],\"side\":\"TOP\"},\"type\":\"ConnectorPlacement.EquallySpacedRectSide\",\"uuid\":\"95ef669c-c6ed-44c3-8b69-447906728b6d\"}]},\"type\":\"ConnectorPlacement.EquallySpacedConnector\",\"uuid\":\"ea66db09-64d7-4d7e-ba7b-d769c56e2dbd\"}],\"packageUris\":[\"http://schema.mathworks.com/mf0/Connector/19700101\"],\"version\":\"1.0\"}"
  EMT SW : Subsystem  VariantControl=EMT_SW
      settings: PortSchema="{\"entries\":[{\"content\":{\"sides\":[{\"content\":{\"connectorIds\":[\"LConn1\",\"LConn2\",\"LConn3\"]},\"type\":\"ConnectorPlacement.EquallySpacedRectSide\",\"uuid\":\"96043b84-a665-4cb2-a938-d6633d7ee474\"},{\"content\":{\"connectorIds\":[\"In1\"],\"side\":\"RIGHT\"},\"type\":\"ConnectorPlacement.EquallySpacedRectSide\",\"uuid\":\"064d463f-c23a-42ac-89ce-8dea3d446214\"},{\"content\":{\"connectorIds\":[],\"side\":\"TOP\"},\"type\":\"ConnectorPlacement.EquallySpacedRectSide\",\"uuid\":\"95ef669c-c6ed-44c3-8b69-447906728b6d\"}]},\"type\":\"ConnectorPlacement.EquallySpacedConnector\",\"uuid\":\"ea66db09-64d7-4d7e-ba7b-d769c56e2dbd\"}],\"packageUris\":[\"http://schema.mathworks.com/mf0/Connector/19700101\"],\"version\":\"1.0\"}"
  Phasor : Subsystem  VariantControl=Phasor
      settings: PortSchema="{\"entries\":[{\"content\":{\"sides\":[{\"content\":{\"connectorIds\":[\"LConn1\",\"LConn2\",\"LConn3\"]},\"type\":\"ConnectorPlacement.EquallySpacedRectSide\",\"uuid\":\"96043b84-a665-4cb2-a938-d6633d7ee474\"},{\"content\":{\"connectorIds\":[\"In1\"],\"side\":\"RIGHT\"},\"type\":\"ConnectorPlacement.EquallySpacedRectSide\",\"uuid\":\"064d463f-c23a-42ac-89ce-8dea3d446214\"},{\"content\":{\"connectorIds\":[],\"side\":\"TOP\"},\"type\":\"ConnectorPlacement.EquallySpacedRectSide\",\"uuid\":\"95ef669c-c6ed-44c3-8b69-447906728b6d\"}]},\"type\":\"ConnectorPlacement.EquallySpacedConnector\",\"uuid\":\"ea66db09-64d7-4d7e-ba7b-d769c56e2dbd\"}],\"packageUris\":[\"http://schema.mathworks.com/mf0/Connector/19700101\"],\"version\":\"1.0\"}"
  A : PMIOPort  Side=Left
  B : PMIOPort  Port=2  Side=Left
  C : PMIOPort  Port=3  Side=Left

== system Scenario_3/G6/VSC/output signals ==
  Vs : Inport
  Is : Inport  Port=2
  control : Inport  Port=3
  Bus Creator : BusCreator  Inputs=15
  Demux : Demux  Outputs=13
  m : Outport
  wires:
  Bus Creator/1 -> m/1
  control/1 -> Demux/1
  Vs/1 -> Bus Creator/1  "Vabc"
  Is/1 -> Bus Creator/2  "Iabc"
  Demux/1 -> Bus Creator/3  "vqp"
  Demux/2 -> Bus Creator/4  "vdp"
  Demux/3 -> Bus Creator/5  "vqn"
  Demux/4 -> Bus Creator/6  "vdn"
  Demux/5 -> Bus Creator/7  "iqp"
  Demux/6 -> Bus Creator/8  "idp"
  Demux/7 -> Bus Creator/9  "iqn"
  Demux/8 -> Bus Creator/10  "idn"
  Demux/9 -> Bus Creator/11  "f"
  Demux/10 -> Bus Creator/12  "Pdq"
  Demux/11 -> Bus Creator/13  "Qdq"
  Demux/12 -> Bus Creator/14  "Pabc"
  Demux/13 -> Bus Creator/15  "Qabc"

== system Scenario_3/G7/VSC/VI measurement ==
  Current Measurement : powerlib/Measurements/Current Measurement  PhasorSimulation=on  OutputType=Complex  PSBequivalent=0
  Current Measurement1 : powerlib/Measurements/Current Measurement  PhasorSimulation=on  OutputType=Complex  PSBequivalent=0
  Current Measurement2 : powerlib/Measurements/Current Measurement  PhasorSimulation=on  OutputType=Complex  PSBequivalent=0
  Ground : powerlib/Elements/Ground  LConnTagsString=a
  Ground1 : powerlib/Elements/Ground  LConnTagsString=a
  Ground2 : powerlib/Elements/Ground  LConnTagsString=a
  Mux : Mux  Inputs=3
  Mux1 : Mux  Inputs=3
  Voltage Measurement : powerlib/Measurements/Voltage Measurement  PhasorSimulation=on  OutputType=Complex  PSBequivalent=0
  Voltage Measurement1 : powerlib/Measurements/Voltage Measurement  PhasorSimulation=on  OutputType=Complex  PSBequivalent=0
  Voltage Measurement2 : powerlib/Measurements/Voltage Measurement  PhasorSimulation=on  OutputType=Complex  PSBequivalent=0
  A : PMIOPort  Side=Left
  B : PMIOPort  Port=2  Side=Left
  C : PMIOPort  Port=3  Side=Left
  a : PMIOPort  Port=4  Side=Right
  b : PMIOPort  Port=5  Side=Right
  c : PMIOPort  Port=6  Side=Right
  Vs : Outport
  Is : Outport  Port=2
  wires:
  Mux1/1 -> Is/1
  Mux/1 -> Vs/1
  Voltage Measurement1/1 -> Mux/2
  Voltage Measurement2/1 -> Mux/3
  Current Measurement2/1 -> Mux1/3
  Voltage Measurement/1 -> Mux/1
  Current Measurement/1 -> Mux1/1
  Current Measurement1/1 -> Mux1/2
  connections:
  Voltage Measurement/LConn1 -- Current Measurement/LConn1 -- A/RConn1
  Current Measurement2/LConn1 -- C/RConn1 -- Voltage Measurement2/LConn1
  Current Measurement1/LConn1 -- Voltage Measurement1/LConn1 -- B/RConn1
  Current Measurement1/RConn1 -- b/RConn1
  Current Measurement/RConn1 -- a/RConn1
  Ground/LConn1 -- Voltage Measurement/LConn2
  Current Measurement2/RConn1 -- c/RConn1
  Ground1/LConn1 -- Voltage Measurement1/LConn2
  Ground2/LConn1 -- Voltage Measurement2/LConn2

== system Scenario_3/G7/VSC/VSC Control ==
  Block : Inport
  Vabc : Inport  Port=2
  Iabc : Inport  Port=3
  Pset : Inport  Port=4
  Qset : Inport  Port=5
  Control loops : Subsystem  Variant=on  VariantControlMode=label  LabelModeActiveChoice=Phasor_I_ref
  Measurements : Subsystem  Variant=on  VariantControlMode=label  LabelModeActiveChoice=Phasor
  Modulation : Subsystem  Variant=on  VariantControlMode=label  LabelModeActiveChoice=Phasor_I_and_PQ
  Mux : Mux  Inputs=2
  Ref : Outport
  m : Outport  Port=2
  wires:
  Control loops/2(iqd+-ref) -> Modulation/3(iqd+-*)
  Control loops/1(vqd+-ref) -> Modulation/2(vqd+-*)
  [PQabc] -> Mux/2
  Measurements/5(PQabc) -> [PQabc]
  Modulation/1(Ref) -> Ref/1
  Measurements/4(theta) -> [theta]
  Vabc/1 -> Measurements/1(Vabc)
  Measurements/1(vqd+-) -> Control loops/3(vqd+-), [vqdpn]
  Measurements/2(iqd+-) -> Control loops/4(iqd+-)
  Measurements/3(freq) -> Control loops/5(freq)
  [theta] -> Modulation/4(theta)
  [vqdpn] -> Modulation/1(vqd+-)
  Iabc/1 -> Measurements/2(Iabc)
  Mux/1 -> m/1
  Control loops/3(m) -> Mux/1
  Pset/1 -> Control loops/1(Pset)
  Qset/1 -> Control loops/2(Qset)
  Block/1 -> Control loops/6(Block)

== system Scenario_3/G7/VSC/VSC Model ==
  Ref : Inport
  EMT AVG : Subsystem  VariantControl=EMT_AVG
      settings: PortSchema="{\"entries\":[{\"content\":{\"sides\":[{\"content\":{\"connectorIds\":[\"LConn1\",\"LConn2\",\"LConn3\"]},\"type\":\"ConnectorPlacement.EquallySpacedRectSide\",\"uuid\":\"96043b84-a665-4cb2-a938-d6633d7ee474\"},{\"content\":{\"connectorIds\":[\"In1\"],\"side\":\"RIGHT\"},\"type\":\"ConnectorPlacement.EquallySpacedRectSide\",\"uuid\":\"064d463f-c23a-42ac-89ce-8dea3d446214\"},{\"content\":{\"connectorIds\":[],\"side\":\"TOP\"},\"type\":\"ConnectorPlacement.EquallySpacedRectSide\",\"uuid\":\"95ef669c-c6ed-44c3-8b69-447906728b6d\"}]},\"type\":\"ConnectorPlacement.EquallySpacedConnector\",\"uuid\":\"ea66db09-64d7-4d7e-ba7b-d769c56e2dbd\"}],\"packageUris\":[\"http://schema.mathworks.com/mf0/Connector/19700101\"],\"version\":\"1.0\"}"
  EMT SW : Subsystem  VariantControl=EMT_SW
      settings: PortSchema="{\"entries\":[{\"content\":{\"sides\":[{\"content\":{\"connectorIds\":[\"LConn1\",\"LConn2\",\"LConn3\"]},\"type\":\"ConnectorPlacement.EquallySpacedRectSide\",\"uuid\":\"96043b84-a665-4cb2-a938-d6633d7ee474\"},{\"content\":{\"connectorIds\":[\"In1\"],\"side\":\"RIGHT\"},\"type\":\"ConnectorPlacement.EquallySpacedRectSide\",\"uuid\":\"064d463f-c23a-42ac-89ce-8dea3d446214\"},{\"content\":{\"connectorIds\":[],\"side\":\"TOP\"},\"type\":\"ConnectorPlacement.EquallySpacedRectSide\",\"uuid\":\"95ef669c-c6ed-44c3-8b69-447906728b6d\"}]},\"type\":\"ConnectorPlacement.EquallySpacedConnector\",\"uuid\":\"ea66db09-64d7-4d7e-ba7b-d769c56e2dbd\"}],\"packageUris\":[\"http://schema.mathworks.com/mf0/Connector/19700101\"],\"version\":\"1.0\"}"
  Phasor : Subsystem  VariantControl=Phasor
      settings: PortSchema="{\"entries\":[{\"content\":{\"sides\":[{\"content\":{\"connectorIds\":[\"LConn1\",\"LConn2\",\"LConn3\"]},\"type\":\"ConnectorPlacement.EquallySpacedRectSide\",\"uuid\":\"96043b84-a665-4cb2-a938-d6633d7ee474\"},{\"content\":{\"connectorIds\":[\"In1\"],\"side\":\"RIGHT\"},\"type\":\"ConnectorPlacement.EquallySpacedRectSide\",\"uuid\":\"064d463f-c23a-42ac-89ce-8dea3d446214\"},{\"content\":{\"connectorIds\":[],\"side\":\"TOP\"},\"type\":\"ConnectorPlacement.EquallySpacedRectSide\",\"uuid\":\"95ef669c-c6ed-44c3-8b69-447906728b6d\"}]},\"type\":\"ConnectorPlacement.EquallySpacedConnector\",\"uuid\":\"ea66db09-64d7-4d7e-ba7b-d769c56e2dbd\"}],\"packageUris\":[\"http://schema.mathworks.com/mf0/Connector/19700101\"],\"version\":\"1.0\"}"
  A : PMIOPort  Side=Left
  B : PMIOPort  Port=2  Side=Left
  C : PMIOPort  Port=3  Side=Left

== system Scenario_3/G7/VSC/output signals ==
  Vs : Inport
  Is : Inport  Port=2
  control : Inport  Port=3
  Bus Creator : BusCreator  Inputs=15
  Demux : Demux  Outputs=13
  m : Outport
  wires:
  Bus Creator/1 -> m/1
  control/1 -> Demux/1
  Vs/1 -> Bus Creator/1  "Vabc"
  Is/1 -> Bus Creator/2  "Iabc"
  Demux/1 -> Bus Creator/3  "vqp"
  Demux/2 -> Bus Creator/4  "vdp"
  Demux/3 -> Bus Creator/5  "vqn"
  Demux/4 -> Bus Creator/6  "vdn"
  Demux/5 -> Bus Creator/7  "iqp"
  Demux/6 -> Bus Creator/8  "idp"
  Demux/7 -> Bus Creator/9  "iqn"
  Demux/8 -> Bus Creator/10  "idn"
  Demux/9 -> Bus Creator/11  "f"
  Demux/10 -> Bus Creator/12  "Pdq"
  Demux/11 -> Bus Creator/13  "Qdq"
  Demux/12 -> Bus Creator/14  "Pabc"
  Demux/13 -> Bus Creator/15  "Qabc"

== system Scenario_3/G9/VSC/VI measurement ==
  Current Measurement : powerlib/Measurements/Current Measurement  PhasorSimulation=on  OutputType=Complex  PSBequivalent=0
  Current Measurement1 : powerlib/Measurements/Current Measurement  PhasorSimulation=on  OutputType=Complex  PSBequivalent=0
  Current Measurement2 : powerlib/Measurements/Current Measurement  PhasorSimulation=on  OutputType=Complex  PSBequivalent=0
  Ground : powerlib/Elements/Ground  LConnTagsString=a
  Ground1 : powerlib/Elements/Ground  LConnTagsString=a
  Ground2 : powerlib/Elements/Ground  LConnTagsString=a
  Mux : Mux  Inputs=3
  Mux1 : Mux  Inputs=3
  Voltage Measurement : powerlib/Measurements/Voltage Measurement  PhasorSimulation=on  OutputType=Complex  PSBequivalent=0
  Voltage Measurement1 : powerlib/Measurements/Voltage Measurement  PhasorSimulation=on  OutputType=Complex  PSBequivalent=0
  Voltage Measurement2 : powerlib/Measurements/Voltage Measurement  PhasorSimulation=on  OutputType=Complex  PSBequivalent=0
  A : PMIOPort  Side=Left
  B : PMIOPort  Port=2  Side=Left
  C : PMIOPort  Port=3  Side=Left
  a : PMIOPort  Port=4  Side=Right
  b : PMIOPort  Port=5  Side=Right
  c : PMIOPort  Port=6  Side=Right
  Vs : Outport
  Is : Outport  Port=2
  wires:
  Mux1/1 -> Is/1
  Mux/1 -> Vs/1
  Voltage Measurement1/1 -> Mux/2
  Voltage Measurement2/1 -> Mux/3
  Current Measurement2/1 -> Mux1/3
  Voltage Measurement/1 -> Mux/1
  Current Measurement/1 -> Mux1/1
  Current Measurement1/1 -> Mux1/2
  connections:
  Voltage Measurement/LConn1 -- Current Measurement/LConn1 -- A/RConn1
  Current Measurement2/LConn1 -- C/RConn1 -- Voltage Measurement2/LConn1
  Current Measurement1/LConn1 -- Voltage Measurement1/LConn1 -- B/RConn1
  Current Measurement1/RConn1 -- b/RConn1
  Current Measurement/RConn1 -- a/RConn1
  Ground/LConn1 -- Voltage Measurement/LConn2
  Current Measurement2/RConn1 -- c/RConn1
  Ground1/LConn1 -- Voltage Measurement1/LConn2
  Ground2/LConn1 -- Voltage Measurement2/LConn2
